simulink model "mechanical"  (Simulink 9.3)
settings: Solver=ode4  StartTime=0  StopTime=500  RelTol=1e-3  EnableMultiTasking=on
undefined symbols (not defined in the file or in its folder): initialconditionxo
libraries: simulink x24, commnoisgen2 x2
settings Model: Creator=Administrator  LastModifiedBy=Shamrooz
settings DataIOCC: LimitDataPoints=on
settings OptimizationCC: ExpressionDepthLimit=2147483647  InitFltsAndDblsToZero=on
settings DebuggingCC: SaveWithParameterizedLinksMsg=none  SignalResolutionControl=TryResolveAllWithWarning  SolverPrmCheckMsg=warning  MultiTaskDSMMsg=warning  MultiTaskCondExecSysMsg=none  StateNameClashWarn=warning
settings GRTTargetCC: TargetFcnLib=ansi_tfl_tmw.mat  GeneratePreprocessorConditionals=Disable all

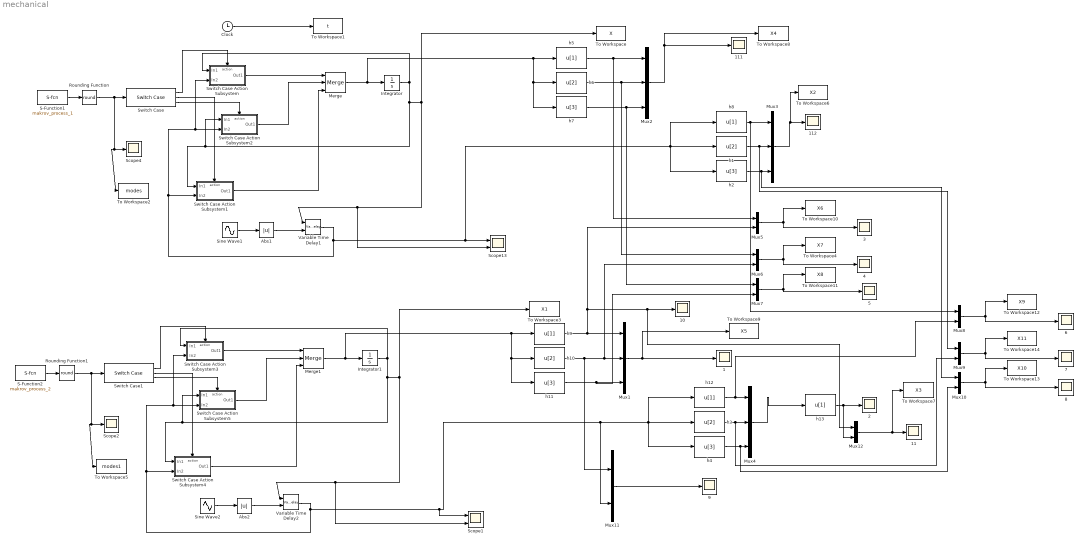
== system mechanical ==
  {1..11,111..112} (13 alike) : Scope
  Abs1 : Abs
  Abs2 : Abs
  Clock : Clock
  Integrator : Integrator  InitialCondition=initialconditionxo
  Integrator1 : Integrator  InitialCondition=[1;-3;5; -7]
  Merge : Merge  Inputs=3
  Merge1 : Merge  Inputs=3
  Mux{1..4} (4 alike) : Mux  Inputs=3
  Mux{5..12} (8 alike) : Mux  Inputs=2
  Rounding Function : Rounding  Operator=round
  Rounding Function1 : Rounding  Operator=round
  S-Function1 : S-Function  FunctionName=makrov_process_1  SFunctionDeploymentMode=off  EnableBusSupport=off
  S-Function2 : S-Function  FunctionName=makrov_process_2  SFunctionDeploymentMode=off  EnableBusSupport=off
  Scope1 : Scope  NumInputPorts=2
  Scope13 : Scope  NumInputPorts=2
  Scope2 : Scope
  Scope4 : Scope
  Sine Wave1 : Sin  Amplitude=1.5  SampleTime=0.01
  Sine Wave2 : Sin  Amplitude=1.5  SampleTime=0.01
  Switch Case : SwitchCase  CaseConditions={1,2,3}  ShowDefaultCase=off
  Switch Case Action Subsystem : Subsystem  TreatAsAtomicUnit=on
  Switch Case Action Subsystem1 : Subsystem  TreatAsAtomicUnit=on
  Switch Case Action Subsystem2 : Subsystem  TreatAsAtomicUnit=on
  Switch Case Action Subsystem3 : Subsystem  TreatAsAtomicUnit=on
  Switch Case Action Subsystem4 : Subsystem  TreatAsAtomicUnit=on
  Switch Case Action Subsystem5 : Subsystem  TreatAsAtomicUnit=on
  Switch Case1 : SwitchCase  CaseConditions={1,2,3}  ShowDefaultCase=off
  To Workspace : ToWorkspace  VariableName=X  SampleTime=-1
  To Workspace1 : ToWorkspace  VariableName=t  SampleTime=-1
  To Workspace10 : ToWorkspace  VariableName=X6  SampleTime=-1
  To Workspace11 : ToWorkspace  VariableName=X8  SampleTime=-1
  To Workspace12 : ToWorkspace  VariableName=X9  SampleTime=-1
  To Workspace13 : ToWorkspace  VariableName=X10  SampleTime=-1
  To Workspace14 : ToWorkspace  VariableName=X11  SampleTime=-1
  To Workspace2 : ToWorkspace  VariableName=modes  SampleTime=-1
  To Workspace3 : ToWorkspace  VariableName=X1  SampleTime=-1
  To Workspace4 : ToWorkspace  VariableName=X7  SampleTime=-1
  To Workspace5 : ToWorkspace  VariableName=modes1  SampleTime=-1
  To Workspace6 : ToWorkspace  VariableName=X2  SampleTime=-1
  To Workspace7 : ToWorkspace  VariableName=X3  SampleTime=-1
  To Workspace8 : ToWorkspace  VariableName=X4  SampleTime=-1
  To Workspace9 : ToWorkspace  VariableName=X5  SampleTime=-1
  Variable Time Delay1 : VariableTransportDelay  MaximumDelay=0.01
  Variable Time Delay2 : VariableTransportDelay  MaximumDelay=0.01
  h{1,3,6,10} (4 alike) : Fcn  Expr=u[2]
  h{2,4,7,11} (4 alike) : Fcn  Expr=u[3]
  h{5,8..9,12..13} (5 alike) : Fcn  Expr=u[1]
  wires:
  Clock/1 -> To Workspace1/1
  S-Function1/1 -> Rounding Function/1
  Switch Case Action Subsystem/1(Out1) -> Merge/1
  Integrator/1 -> Switch Case Action Subsystem/1(In1), To Workspace/1, Variable Time Delay1/1, Scope13/2, Switch Case Action Subsystem1/1(In1), Switch Case Action Subsystem2/1(In1)
  Switch Case/1 -> Switch Case Action Subsystem/Action
  Switch Case/2 -> Switch Case Action Subsystem1/Action
  Rounding Function/1 -> Switch Case/1, Scope4/1, To Workspace2/1
  Abs1/1 -> Variable Time Delay1/2
  Variable Time Delay1/1 -> Switch Case Action Subsystem1/2(In2), Switch Case Action Subsystem/2(In2), Switch Case Action Subsystem2/2(In2), h8/1, h2/1, h1/1, Scope13/1
  Sine Wave1/1 -> Abs1/1
  Switch Case/3 -> Switch Case Action Subsystem2/Action
  Switch Case Action Subsystem2/1(Out1) -> Merge/2
  Switch Case Action Subsystem1/1(Out1) -> Merge/3
  Merge/1 -> h7/1, h6/1, h5/1, Integrator/1
  Mux2/1 -> To Workspace8/1, 111/1
  h7/1 -> Mux7/1, Mux2/3
  Mux3/1 -> To Workspace6/1, 112/1
  h8/1 -> Mux8/1, Mux3/1
  h1/1 -> Mux9/1, Mux3/2
  h2/1 -> Mux10/1, Mux3/3
  h5/1 -> Mux5/1, Mux2/1
  Mux5/1 -> 3/1, To Workspace10/1
  S-Function2/1 -> Rounding Function1/1
  Switch Case Action Subsystem3/1(Out1) -> Merge1/1
  Integrator1/1 -> Switch Case Action Subsystem3/1(In1), To Workspace3/1, Variable Time Delay2/1, Scope1/2, Switch Case Action Subsystem4/1(In1), Switch Case Action Subsystem5/1(In1)
  Switch Case1/1 -> Switch Case Action Subsystem3/Action
  Switch Case1/2 -> Switch Case Action Subsystem4/Action
  Rounding Function1/1 -> Switch Case1/1, Scope2/1, To Workspace5/1
  Abs2/1 -> Variable Time Delay2/2
  Variable Time Delay2/1 -> Switch Case Action Subsystem4/2(In2), Switch Case Action Subsystem3/2(In2), Switch Case Action Subsystem5/2(In2), h12/1, h4/1, h3/1, Mux11/2, Scope1/1
  Sine Wave2/1 -> Abs2/1
  Switch Case1/3 -> Switch Case Action Subsystem5/Action
  Switch Case Action Subsystem5/1(Out1) -> Merge1/2
  Switch Case Action Subsystem4/1(Out1) -> Merge1/3
  Merge1/1 -> h11/1, h10/1, h9/1, Integrator1/1
  Mux1/1 -> To Workspace9/1, 1/1
  h10/1 -> Mux11/1, Mux6/2, Mux1/2
  h11/1 -> Mux7/2, Mux1/3
  Mux4/1 -> h13/1
  h12/1 -> Mux8/2, Mux4/1
  h3/1 -> Mux9/2, Mux4/2
  h4/1 -> Mux10/2, Mux4/3
  h9/1 -> Mux1/1, Mux12/1, 10/1, Mux5/2
  Mux6/1 -> 4/1, To Workspace4/1
  h6/1 -> Mux6/1, Mux2/2
  Mux7/1 -> 5/1, To Workspace11/1
  Mux8/1 -> 6/1, To Workspace12/1
  Mux9/1 -> 7/1, To Workspace14/1
  Mux10/1 -> 8/1, To Workspace13/1
  Mux11/1 -> 9/1
  h13/1 -> Mux12/2, 2/1
  Mux12/1 -> To Workspace7/1, 11/1

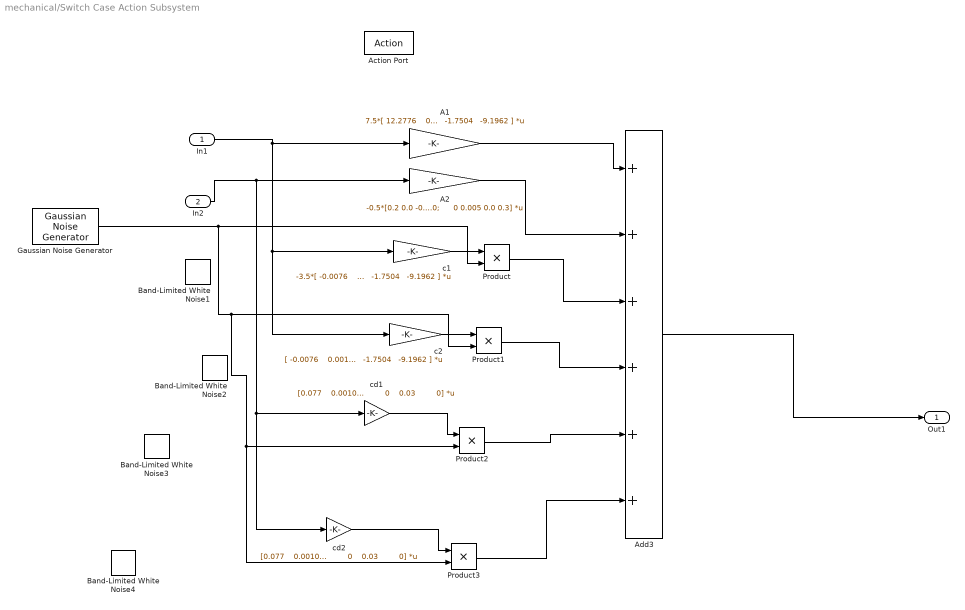
== system mechanical/Switch Case Action Subsystem ==
  In1 : Inport
  In2 : Inport  Port=2
  Action Port : ActionPort  ActionPortLabel=case [ 1 ]:
  A1 : Gain  Gain=|  Multiplication=Matrix(K*u) (u vector)
      | 7.5*[ 12.2776    0.0105   -0.0298   -0.4748;
      |     0.0189   0.2205    0.0554    7.9508;
      |     0.3689   -0.0259   -5.4261   1.6897;
      |     0         0    1.0000         0  ]+[12.3   ; 6.2 ; 4.3; -15.5]*[   -21.4018   -3.6824   -1.7504   -9.1962
      | ]
  A2 : Gain  Gain=|  Multiplication=Matrix(K*u) (u vector)
      | -0.5*[0.2 0.0 -0.002 0;
      |     0 0.5 0.004 -0.003;
      |     -0.007 0.3 0.02 0; 
      |     0 0.005 0.0 0.3]
  Add3 : Sum  Inputs=++++++
  Band-Limited White Noise{1..4} (4 alike) : simulink/Sources/Band-Limited White Noise  Cov=[3.9]  Ts=0.01  seed=[23341]
  Gaussian Noise Generator : commnoisgen2/Gaussian Noise Generator  m=0.5  d=5  s=67  Ts=0.01  frameBased=off  sampPerFrame=1  orient=off  outDataType=double
      link override Constant: OutDataTypeStr=double
      settings: SourceProductName=Communications Toolbox  SourceProductBaseCode=CM
  Product{,1..3} (4 alike) : Product  RndMeth=Zero
  c1 : Gain  Gain=|  Multiplication=Matrix(K*u) (u vector)
      | -3.5*[ -0.0076    0.0015   -0.0029   -0.0047;
      |     0.0018   -0.0025    0.0055    0.00158;
      |     0.00368   -0.00259   -0.00426   -0.00189;
      |          0         0    0.003         0]+[0.002   ; -0.003 ; 0.005; 0.003]*[   -21.4018   -3.6824   -1.7504   -9.1962
      | ]
  c2 : Gain  Gain=|  Multiplication=Matrix(K*u) (u vector)
      | [ -0.0076    0.0015   -0.0029   -0.0047;
      |     0.0018   -0.0025    0.0055    0.00158;
      |     0.00368   -0.00259   -0.00426   -0.00189;
      |          0         0    0.003         0]+[0.002   ; -0.003 ; 0.005; 0.003]*[  -21.4018   -3.6824   -1.7504   -9.1962
      | ]
  cd1 : Gain  Gain=|  Multiplication=Matrix(K*u) (u vector)
      | [0.077    0.00105   -0.0029   -0.0047;
      |     0.0018   0.022    0.0055    0.0951;
      |     0.0036   -0.0025   0.042   -0.0068;
      |          0         0    0.03         0]
  cd2 : Gain  Gain=|  Multiplication=Matrix(K*u) (u vector)
      | [0.077    0.00105   -0.0029   -0.0047;
      |     0.0018   0.022    0.0055    0.0951;
      |     0.0036   -0.0025   0.042   -0.0068;
      |          0         0    0.03         0]
  Out1 : Outport
  wires:
  In1/1 -> A1/1, c1/1, c2/1
  In2/1 -> A2/1, cd1/1, cd2/1
  A1/1 -> Add3/1
  c1/1 -> Product/1
  c2/1 -> Product1/1
  cd1/1 -> Product2/1
  cd2/1 -> Product3/1
  A2/1 -> Add3/2
  Product/1 -> Add3/3
  Product1/1 -> Add3/4
  Product2/1 -> Add3/5
  Product3/1 -> Add3/6
  Add3/1 -> Out1/1
  Gaussian Noise Generator/1 -> Product/2, Product3/2, Product2/2, Product1/2

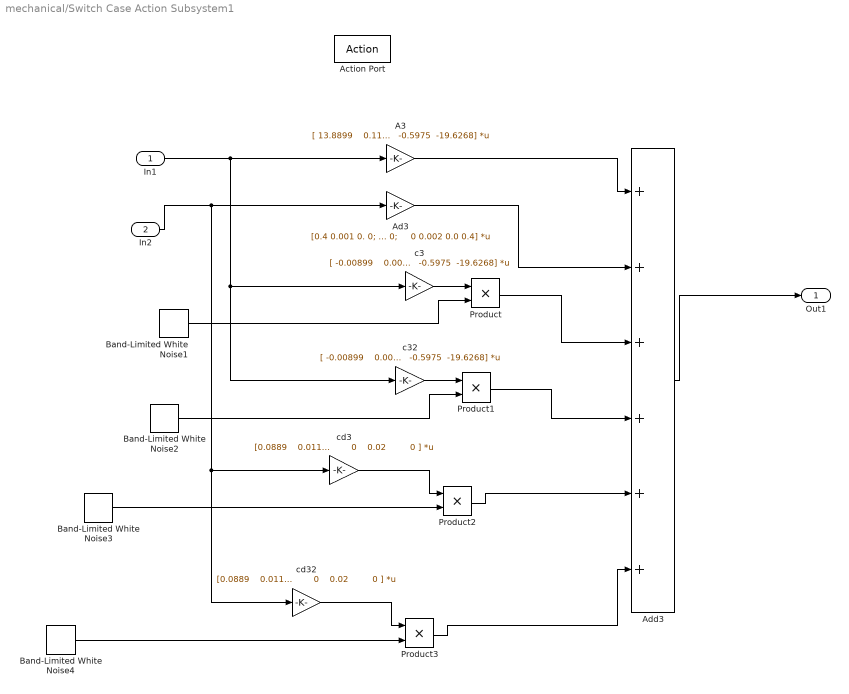
== system mechanical/Switch Case Action Subsystem1 ==
  In1 : Inport
  In2 : Inport  Port=2
  Action Port : ActionPort  ActionPortLabel=case [ 2 ]:
  A3 : Gain  Gain=|  Multiplication=Matrix(K*u) (u vector)
      | [ 13.8899    0.1164    0.1239    0.3561;
      |     0.7474    0.8768    3.1617   2.0275;
      |     3.4031   -1.8410   -7.3748  18.0287;
      |       0         0    1.0000       0
      | ]+[12.4   ; 6.4 ; 4.6; -17.6]*[    -31.4271   -3.4304   -0.5975  -19.6268]
  Ad3 : Gain  Gain=|  Multiplication=Matrix(K*u) (u vector)
      | [0.4 0.001 0. 0;
      |     0 0.3 0.002 -0.003;
      |     -0.004 0.3 0.02 0;
      |     0 0.002 0.0 0.4]
  Add3 : Sum  Inputs=++++++
  Band-Limited White Noise{1..4} (4 alike) : simulink/Sources/Band-Limited White Noise  Cov=[3.9]  Ts=0.01  seed=[23341]
  Product{,1..3} (4 alike) : Product  RndMeth=Zero
  c3 : Gain  Gain=|  Multiplication=Matrix(K*u) (u vector)
      | [ -0.00899    0.001164    0.001239    0.00356;
      |     0.00747    -0.001768    0.001617   0.00275;
      |     0.00403   -0.00841   -0.003748  -0.00287;
      |              0         0    0.002         0
      | ]+[0.004   ; -0.005 ; 0.007; 0.008]*[    -31.4271   -3.4304   -0.5975  -19.6268]
  c32 : Gain  Gain=|  Multiplication=Matrix(K*u) (u vector)
      | [ -0.00899    0.001164    0.001239    0.00356;
      |     0.00747    -0.001768    0.001617   0.00275;
      |     0.00403   -0.00841   -0.003748  -0.00287;
      |              0         0    0.002         0
      | ]+[0.004   ; -0.005 ; 0.007; 0.008]*[   -31.4271   -3.4304   -0.5975  -19.6268]
  cd3 : Gain  Gain=|  Multiplication=Matrix(K*u) (u vector)
      | [0.0889    0.0116    0.0123    0.0356;
      |     0.0074   0.0176   0.0161   0.0027;
      |     0.0403   -0.0084   0.0374  -0.0028;
      |       0         0    0.02         0
      | ]
  cd32 : Gain  Gain=|  Multiplication=Matrix(K*u) (u vector)
      | [0.0889    0.0116    0.0123    0.0356;
      |     0.0074   0.0176   0.0161   0.0027;
      |     0.0403   -0.0084   0.0374  -0.0028;
      |       0         0    0.02         0
      | ]
  Out1 : Outport
  wires:
  In1/1 -> A3/1, c3/1, c32/1
  Add3/1 -> Out1/1
  In2/1 -> Ad3/1, cd3/1, cd32/1
  A3/1 -> Add3/1
  c3/1 -> Product/1
  Band-Limited White Noise1/1 -> Product/2
  Ad3/1 -> Add3/2
  Product/1 -> Add3/3
  c32/1 -> Product1/1
  Band-Limited White Noise2/1 -> Product1/2
  Product1/1 -> Add3/4
  cd3/1 -> Product2/1
  Band-Limited White Noise3/1 -> Product2/2
  Product2/1 -> Add3/5
  cd32/1 -> Product3/1
  Band-Limited White Noise4/1 -> Product3/2
  Product3/1 -> Add3/6

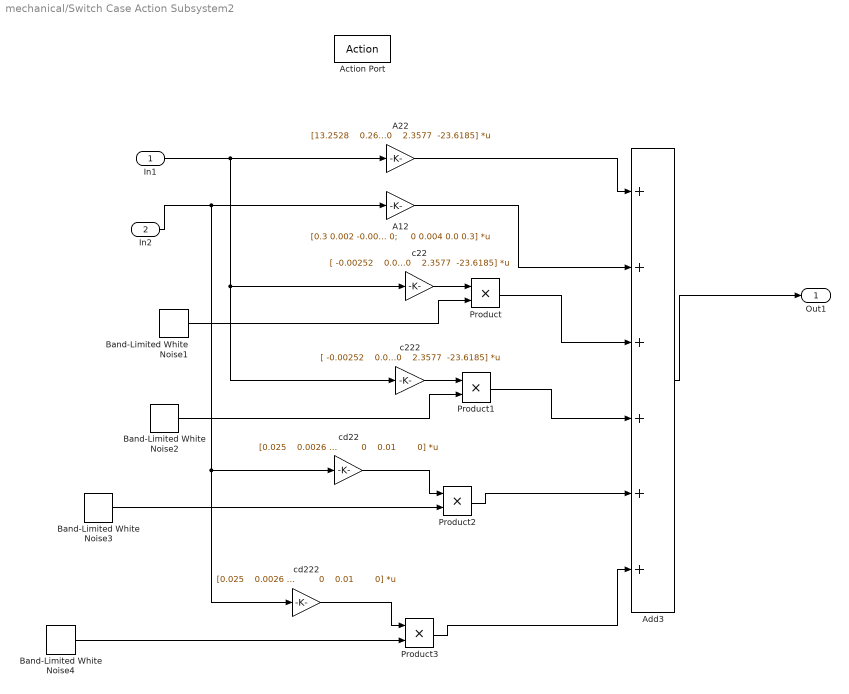
== system mechanical/Switch Case Action Subsystem2 ==
  In1 : Inport
  In2 : Inport  Port=2
  Action Port : ActionPort  ActionPortLabel=case [ 3 ]:
  A12 : Gain  Gain=|  Multiplication=Matrix(K*u) (u vector)
      | [0.3 0.002 -0.001 0;
      |     0 0.3 0.0 -0.003;
      |     -0.0 0.3 0.02 0;
      |     0 0.004 0.0 0.3]
  A22 : Gain  Gain=|  Multiplication=Matrix(K*u) (u vector)
      | [13.2528    0.2688    0.0454   -0.1692;
      |    -0.8758   0.6408    1.3903    7.8546;
      |     3.1426   -1.8312   -6.1510   6.6448;
      |      0         0    1.0000         0  ]+[12.5   ; 6.3 ; 4.5; -16.4]*[  -48.3874   -4.8260    2.3577  -23.6185]
  Add3 : Sum  Inputs=++++++
  Band-Limited White Noise{1..4} (4 alike) : simulink/Sources/Band-Limited White Noise  Cov=[3.9]  Ts=0.01  seed=[23341]
  Product{,1..3} (4 alike) : Product  RndMeth=Zero
  c22 : Gain  Gain=|  Multiplication=Matrix(K*u) (u vector)
      | [ -0.00252    0.00268    0.00454   -0.0169;
      |    -0.00875   -0.00148    0.00393    0.00154;
      |     0.00142   -0.00132   -0.00151   -0.00144;
      |          0         0    0.001        0]+[0.003   ; -0.004 ; 0.006; 0.007]*[  -48.3874   -4.8260    2.3577  -23.6185]
  c222 : Gain  Gain=|  Multiplication=Matrix(K*u) (u vector)
      | [ -0.00252    0.00268    0.00454   -0.0169;
      |    -0.00875   -0.00148    0.00393    0.00154;
      |     0.00142   -0.00132   -0.00151   -0.00144;
      |          0         0    0.001        0]+[0.003   ; -0.004 ; 0.006; 0.007]*[  -48.3874   -4.8260    2.3577  -23.6185]
  cd22 : Gain  Gain=|  Multiplication=Matrix(K*u) (u vector)
      | [0.025    0.0026    0.0045   -0.0016;
      |    -0.0087   0.0641    0.0392    0.0085;
      |     0.0142  -0.0831  0.0151   -0.0644;
      |      0         0    0.01        0]
  cd222 : Gain  Gain=|  Multiplication=Matrix(K*u) (u vector)
      | [0.025    0.0026    0.0045   -0.0016;
      |    -0.0087   0.0641    0.0392    0.0085;
      |     0.0142  -0.0831  0.0151   -0.0644;
      |      0         0    0.01        0]
  Out1 : Outport
  wires:
  In1/1 -> A22/1, c22/1, c222/1
  Add3/1 -> Out1/1
  In2/1 -> A12/1, cd22/1, cd222/1
  A22/1 -> Add3/1
  c22/1 -> Product/1
  Band-Limited White Noise1/1 -> Product/2
  A12/1 -> Add3/2
  Product/1 -> Add3/3
  c222/1 -> Product1/1
  Band-Limited White Noise2/1 -> Product1/2
  Product1/1 -> Add3/4
  cd22/1 -> Product2/1
  Band-Limited White Noise3/1 -> Product2/2
  Product2/1 -> Add3/5
  cd222/1 -> Product3/1
  Band-Limited White Noise4/1 -> Product3/2
  Product3/1 -> Add3/6

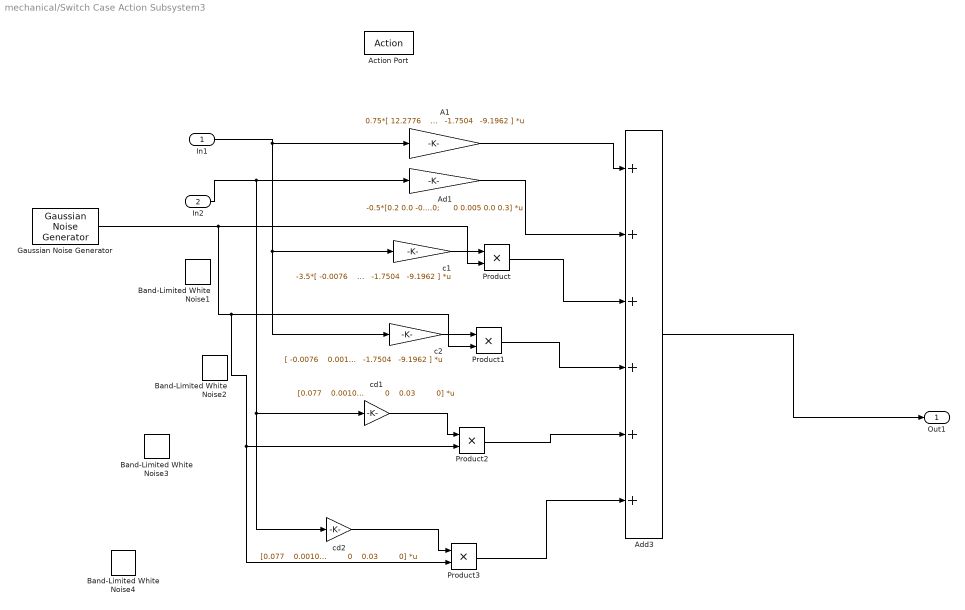
== system mechanical/Switch Case Action Subsystem3 ==
  In1 : Inport
  In2 : Inport  Port=2
  Action Port : ActionPort  ActionPortLabel=case [ 1 ]:
  A1 : Gain  Gain=|  Multiplication=Matrix(K*u) (u vector)
      | 0.75*[ 12.2776    0.0105   -0.0298   -0.4748;
      |     0.0189   0.2205    0.0554    7.9508;
      |     0.3689   -0.0259   -5.4261   1.6897;
      |     0         0    1.0000         0  ]+[12.3   ; 6.2 ; 4.3; -15.5]*[   -21.4018   -3.6824   -1.7504   -9.1962
      | ]
  Ad1 : Gain  Gain=|  Multiplication=Matrix(K*u) (u vector)
      | -0.5*[0.2 0.0 -0.002 0;
      |     0 0.5 0.004 -0.003;
      |     -0.007 0.3 0.02 0; 
      |     0 0.005 0.0 0.3]
  Add3 : Sum  Inputs=++++++
  Band-Limited White Noise{1..4} (4 alike) : simulink/Sources/Band-Limited White Noise  Cov=[3.9]  Ts=0.01  seed=[23341]
  Gaussian Noise Generator : commnoisgen2/Gaussian Noise Generator  m=0.5  d=5  s=67  Ts=0.01  frameBased=off  sampPerFrame=1  orient=off  outDataType=double
      link override Constant: OutDataTypeStr=double
      settings: SourceProductName=Communications Toolbox  SourceProductBaseCode=CM
  Product{,1..3} (4 alike) : Product  RndMeth=Zero
  c1 : Gain  Gain=|  Multiplication=Matrix(K*u) (u vector)
      | -3.5*[ -0.0076    0.0015   -0.0029   -0.0047;
      |     0.0018   -0.0025    0.0055    0.00158;
      |     0.00368   -0.00259   -0.00426   -0.00189;
      |          0         0    0.003         0]+[0.002   ; -0.003 ; 0.005; 0.003]*[   -21.4018   -3.6824   -1.7504   -9.1962
      | ]
  c2 : Gain  Gain=|  Multiplication=Matrix(K*u) (u vector)
      | [ -0.0076    0.0015   -0.0029   -0.0047;
      |     0.0018   -0.0025    0.0055    0.00158;
      |     0.00368   -0.00259   -0.00426   -0.00189;
      |          0         0    0.003         0]+[0.002   ; -0.003 ; 0.005; 0.003]*[  -21.4018   -3.6824   -1.7504   -9.1962
      | ]
  cd1 : Gain  Gain=|  Multiplication=Matrix(K*u) (u vector)
      | [0.077    0.00105   -0.0029   -0.0047;
      |     0.0018   0.022    0.0055    0.0951;
      |     0.0036   -0.0025   0.042   -0.0068;
      |          0         0    0.03         0]
  cd2 : Gain  Gain=|  Multiplication=Matrix(K*u) (u vector)
      | [0.077    0.00105   -0.0029   -0.0047;
      |     0.0018   0.022    0.0055    0.0951;
      |     0.0036   -0.0025   0.042   -0.0068;
      |          0         0    0.03         0]
  Out1 : Outport
  wires:
  In1/1 -> A1/1, c1/1, c2/1
  In2/1 -> Ad1/1, cd1/1, cd2/1
  A1/1 -> Add3/1
  c1/1 -> Product/1
  c2/1 -> Product1/1
  cd1/1 -> Product2/1
  cd2/1 -> Product3/1
  Ad1/1 -> Add3/2
  Product/1 -> Add3/3
  Product1/1 -> Add3/4
  Product2/1 -> Add3/5
  Product3/1 -> Add3/6
  Add3/1 -> Out1/1
  Gaussian Noise Generator/1 -> Product/2, Product3/2, Product2/2, Product1/2

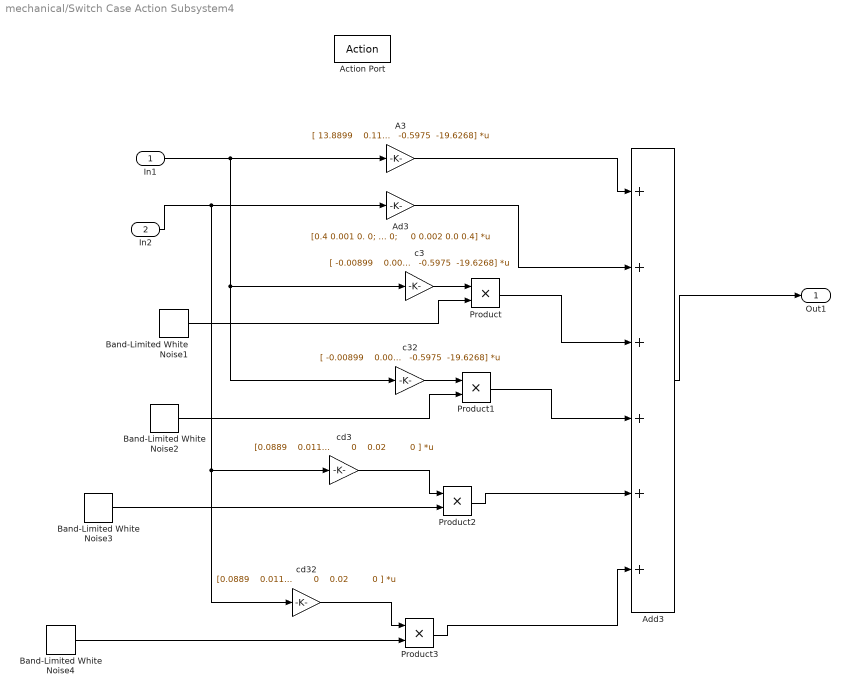
== system mechanical/Switch Case Action Subsystem4 ==
  In1 : Inport
  In2 : Inport  Port=2
  Action Port : ActionPort  ActionPortLabel=case [ 2 ]:
  A3 : Gain  Gain=|  Multiplication=Matrix(K*u) (u vector)
      | [ 13.8899    0.1164    0.1239    0.3561;
      |     0.7474    0.8768    3.1617   2.0275;
      |     3.4031   -1.8410   -7.3748  18.0287;
      |       0         0    1.0000       0
      | ]+[12.4   ; 6.4 ; 4.6; -17.6]*[    -31.4271   -3.4304   -0.5975  -19.6268]
  Ad3 : Gain  Gain=|  Multiplication=Matrix(K*u) (u vector)
      | [0.4 0.001 0. 0;
      |     0 0.3 0.002 -0.003;
      |     -0.004 0.3 0.02 0;
      |     0 0.002 0.0 0.4]
  Add3 : Sum  Inputs=++++++
  Band-Limited White Noise{1..4} (4 alike) : simulink/Sources/Band-Limited White Noise  Cov=[3.9]  Ts=0.01  seed=[23341]
  Product{,1..3} (4 alike) : Product  RndMeth=Zero
  c3 : Gain  Gain=|  Multiplication=Matrix(K*u) (u vector)
      | [ -0.00899    0.001164    0.001239    0.00356;
      |     0.00747    -0.001768    0.001617   0.00275;
      |     0.00403   -0.00841   -0.003748  -0.00287;
      |              0         0    0.002         0
      | ]+[0.004   ; -0.005 ; 0.007; 0.008]*[    -31.4271   -3.4304   -0.5975  -19.6268]
  c32 : Gain  Gain=|  Multiplication=Matrix(K*u) (u vector)
      | [ -0.00899    0.001164    0.001239    0.00356;
      |     0.00747    -0.001768    0.001617   0.00275;
      |     0.00403   -0.00841   -0.003748  -0.00287;
      |              0         0    0.002         0
      | ]+[0.004   ; -0.005 ; 0.007; 0.008]*[   -31.4271   -3.4304   -0.5975  -19.6268]
  cd3 : Gain  Gain=|  Multiplication=Matrix(K*u) (u vector)
      | [0.0889    0.0116    0.0123    0.0356;
      |     0.0074   0.0176   0.0161   0.0027;
      |     0.0403   -0.0084   0.0374  -0.0028;
      |       0         0    0.02         0
      | ]
  cd32 : Gain  Gain=|  Multiplication=Matrix(K*u) (u vector)
      | [0.0889    0.0116    0.0123    0.0356;
      |     0.0074   0.0176   0.0161   0.0027;
      |     0.0403   -0.0084   0.0374  -0.0028;
      |       0         0    0.02         0
      | ]
  Out1 : Outport
  wires:
  In1/1 -> A3/1, c3/1, c32/1
  Add3/1 -> Out1/1
  In2/1 -> Ad3/1, cd3/1, cd32/1
  A3/1 -> Add3/1
  c3/1 -> Product/1
  Band-Limited White Noise1/1 -> Product/2
  Ad3/1 -> Add3/2
  Product/1 -> Add3/3
  c32/1 -> Product1/1
  Band-Limited White Noise2/1 -> Product1/2
  Product1/1 -> Add3/4
  cd3/1 -> Product2/1
  Band-Limited White Noise3/1 -> Product2/2
  Product2/1 -> Add3/5
  cd32/1 -> Product3/1
  Band-Limited White Noise4/1 -> Product3/2
  Product3/1 -> Add3/6

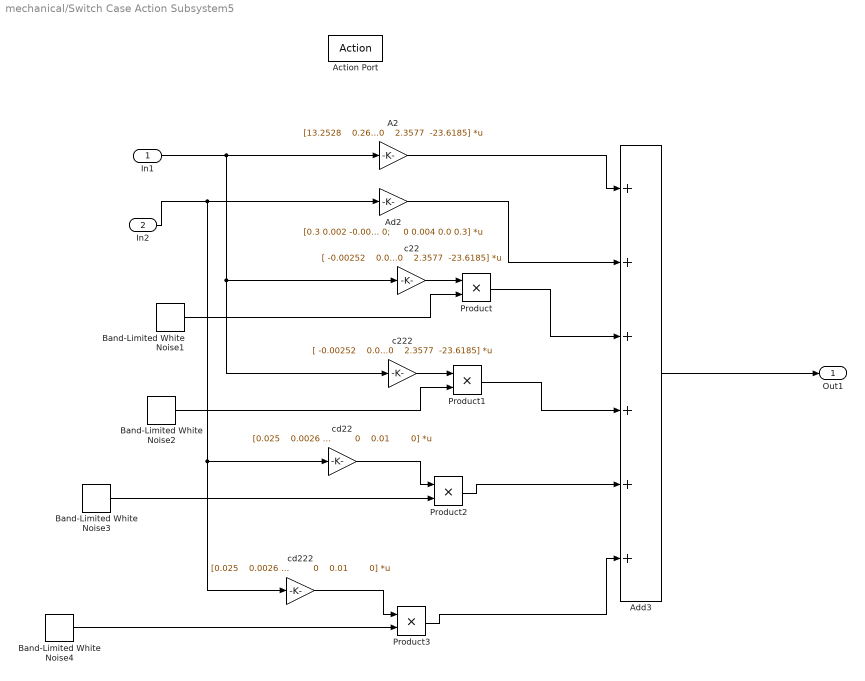
== system mechanical/Switch Case Action Subsystem5 ==
  In1 : Inport
  In2 : Inport  Port=2
  Action Port : ActionPort  ActionPortLabel=case [ 3 ]:
  A2 : Gain  Gain=|  Multiplication=Matrix(K*u) (u vector)
      | [13.2528    0.2688    0.0454   -0.1692;
      |    -0.8758   0.6408    1.3903    7.8546;
      |     3.1426   -1.8312   -6.1510   6.6448;
      |      0         0    1.0000         0  ]+[12.5   ; 6.3 ; 4.5; -16.4]*[  -48.3874   -4.8260    2.3577  -23.6185]
  Ad2 : Gain  Gain=|  Multiplication=Matrix(K*u) (u vector)
      | [0.3 0.002 -0.001 0;
      |     0 0.3 0.0 -0.003;
      |     -0.0 0.3 0.02 0;
      |     0 0.004 0.0 0.3]
  Add3 : Sum  Inputs=++++++
  Band-Limited White Noise{1..4} (4 alike) : simulink/Sources/Band-Limited White Noise  Cov=[3.9]  Ts=0.01  seed=[23341]
  Product{,1..3} (4 alike) : Product  RndMeth=Zero
  c22 : Gain  Gain=|  Multiplication=Matrix(K*u) (u vector)
      | [ -0.00252    0.00268    0.00454   -0.0169;
      |    -0.00875   -0.00148    0.00393    0.00154;
      |     0.00142   -0.00132   -0.00151   -0.00144;
      |          0         0    0.001        0]+[0.003   ; -0.004 ; 0.006; 0.007]*[  -48.3874   -4.8260    2.3577  -23.6185]
  c222 : Gain  Gain=|  Multiplication=Matrix(K*u) (u vector)
      | [ -0.00252    0.00268    0.00454   -0.0169;
      |    -0.00875   -0.00148    0.00393    0.00154;
      |     0.00142   -0.00132   -0.00151   -0.00144;
      |          0         0    0.001        0]+[0.003   ; -0.004 ; 0.006; 0.007]*[  -48.3874   -4.8260    2.3577  -23.6185]
  cd22 : Gain  Gain=|  Multiplication=Matrix(K*u) (u vector)
      | [0.025    0.0026    0.0045   -0.0016;
      |    -0.0087   0.0641    0.0392    0.0085;
      |     0.0142  -0.0831  0.0151   -0.0644;
      |      0         0    0.01        0]
  cd222 : Gain  Gain=|  Multiplication=Matrix(K*u) (u vector)
      | [0.025    0.0026    0.0045   -0.0016;
      |    -0.0087   0.0641    0.0392    0.0085;
      |     0.0142  -0.0831  0.0151   -0.0644;
      |      0         0    0.01        0]
  Out1 : Outport
  wires:
  In1/1 -> A2/1, c22/1, c222/1
  Add3/1 -> Out1/1
  In2/1 -> Ad2/1, cd22/1, cd222/1
  A2/1 -> Add3/1
  c22/1 -> Product/1
  Band-Limited White Noise1/1 -> Product/2
  Ad2/1 -> Add3/2
  Product/1 -> Add3/3
  c222/1 -> Product1/1
  Band-Limited White Noise2/1 -> Product1/2
  Product1/1 -> Add3/4
  cd22/1 -> Product2/1
  Band-Limited White Noise3/1 -> Product2/2
  Product2/1 -> Add3/5
  cd222/1 -> Product3/1
  Band-Limited White Noise4/1 -> Product3/2
  Product3/1 -> Add3/6
